simulink model "Experiment_134_cs"  (Simulink 10.1)
settings: Solver=ode8  StartTime=0.0  StopTime=20  FixedStep=1/10  RelTol=1e-3
PreLoadFcn:
  | mbxruntime.callbacks.PreLoadFcn(bdroot);
PostLoadFcn:
  | mbxruntime.callbacks.PostLoadFcn(bdroot);
InitFcn:
  | mbxruntime.callbacks.InitFcn(bdroot);
StartFcn:
  | mbxruntime.callbacks.StartFcn(bdroot);
StopFcn:
  | mbxruntime.callbacks.StopFcn(bdroot);
undefined symbols (not defined in the file or in its folder): acce_1, acce_2, acce_3, brake, steer, steer_1, steer_2, steer_3, t0_1, t0_2, t0_3, throttle, v_1, v_2, v_3, v_4
libraries: simulink x79, simulink_extras x12, PreScanSimulinkLibrary x8
(part 2 of 9)

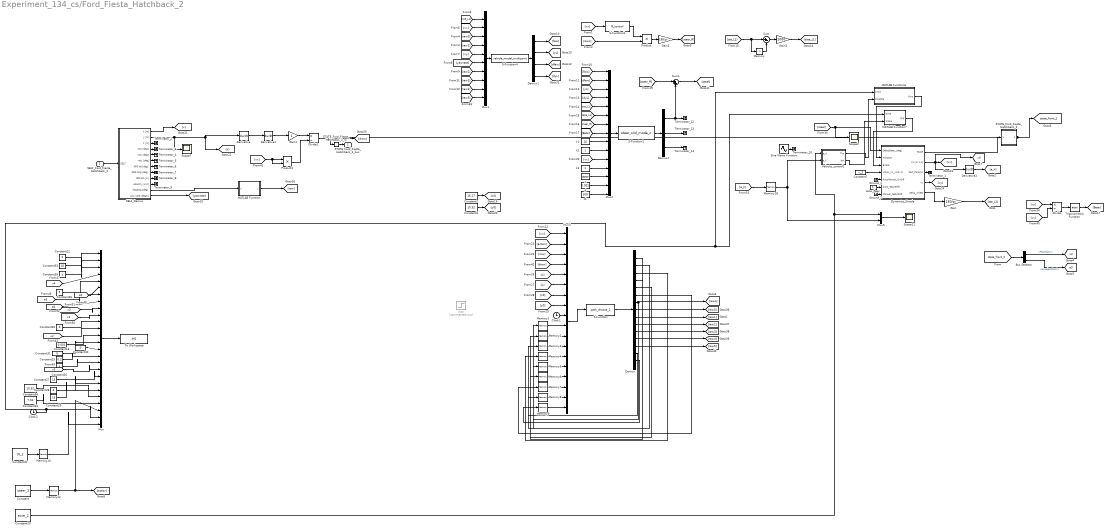
== system Experiment_134_cs/Ford_Fiesta_Hatchback_2 ==
  SELF_Ford_Fiesta_Hatchback_2 : Inport  Tag=inport/SelfPort  OutDataTypeStr=Bus: PRESCAN_SELFSENSORDATA  PortDimensions=1  SampleTime=1/10  BusOutputAsStruct=on
  Auto_Gear : Constant  Tag=AutoGear
  Bus Selector : BusSelector  OutputSignals=PositionX,AccelerationX
  Clock1 : Clock
  Clock2 : Clock
  Constant : Constant  Value=steer_2
  Constant18 : Constant  Value=0.001
  Constant2 : Constant  Value=16.27
  Constant20 : Constant  Value=acce_2
  Constant21 : Constant  Value=t0_2
  Constant22 : Constant  Value=3
  Constant25 : Constant  Value=0.2
  Constant26 : Constant  Value=6
  Constant27 : Constant  Value=15
  Constant28 : Constant  Value=4
  Constant29 : Constant  Value=15
  Constant3 : Constant  Value=10.52
  Constant30 : Constant  Value=0
  Constant31 : Constant  Value=0
  Constant32 : Constant  Value=7.04
  Constant33 : Constant  Value=10
  Constant34 : Constant  Value=10.52
  Constant35 : Constant
  Constant36 : Constant  Value=5
  Constant40 : Constant  Value=0
  Constant7 : Constant  Value=v_3
  Demux : Demux  Outputs=15
  Demux1 : Demux
  Demux2 : Demux  Outputs=3
  Derivative : Derivative
  Derivative1 : Derivative
  Derivative2 : Derivative
  Divide : Product  Inputs=*/
  Divide1 : Product  Inputs=*/
  Dynamics_Simple : Subsystem  Tag=Simple_Vehicle_Dynamics  mask(PreScan Block: Simple Dynamics){Migrate=on, TimeStep=1/10, ComputationMode=Continuous_Time}
      mask prompts: Migrate "Migrate. During migration this block will be replaced by a newer one."; TimeStep "Auto assigned: Time Step [s]"; ComputationMode "Computation mode:"
      mask help:
      | The Simple Dynamics Model is selected in the GUI to simulate vehicle dynamics behavior.
      |
      | The Simple Dynamics Model is completely open to the user. The parameters of this model can be set in the Simple Dynamics dialog in the GUI.
      |
      | For more information, please click Help.
      mask init:
      | p = SimpleDyn_pars;
      settings: DeleteFcn=PreScanBlockDeleteFcn;
      mask Help: eval('openHelp(220)')
      mask Display:
      | image(imread('SimpleDyn.png'))
      | port_label('input', 1, '{\delta}_S_t_ _e_e_r [deg]','texmode','on')
      | port_label('input', 2, 'Throttle [%]')
      | port_label('input', 3, 'Brake Pres [bar]')
      | port_label('input', 4, 'V_0 [ms-1]','texmode','on')
      | port_label('input', 5, 'Auto=[0]/Manual=[1]')
      | port_label('input', 6, 'Auto_GearShift')
      | port_label('input', 7, 'Manual_GearShift')
      | port_label('output', 1, 'State')
      | port_label('output', 2, 'Vx [ms-1]')
      | port_label('output', 3, 'Perf Params')
  Gain : Gain  Gain=180/pi
  Gain1 : Gain
  Gain2 : Gain  Gain=180/pi
  Gain3 : Gain  Gain=1000
  Ground_1 : Ground
  Ground_2 : Ground
  MATLAB Function : MATLAB Function  TreatAsAtomicUnit=on
  MATLAB Function6 : MATLAB Function  TreatAsAtomicUnit=on
  MATLAB Function7 : MATLAB Function  TreatAsAtomicUnit=on
  Memory{,1..9,18} (11 alike) : Memory
  Memory10 : Memory  InitialCondition=-3
  Memory12 : Memory  InitialCondition=10.52
  Mux : Mux  Inputs=26
  Mux1 : Mux  Inputs=10
  Mux2 : Mux  Inputs=15
  Mux3 : Mux  Inputs=18
  Mux5 : Mux  Inputs=2
  Product : Product
  Product1 : Product
  S-Function : S-Function  FunctionName=path_choose_2  SFunctionDeploymentMode=off  EnableBusSupport=off
  S-Function1 : S-Function  FunctionName=steer_slid_mode_c  SFunctionDeploymentMode=off  EnableBusSupport=off
  S-Function3 : S-Function  FunctionName=ff_control  SFunctionDeploymentMode=off  EnableBusSupport=off
  S-Function4 : S-Function  FunctionName=vehicle_model_multipoint  SFunctionDeploymentMode=off  EnableBusSupport=off
  SELF_Demux : Subsystem  Tag=demux/SelfPort  mask(PreScan Demux Block:){}
      mask help:
      | The SELF port shows (state) information of the actor itself. The outputs are position in the experiment's axis system and the GPS coordinates, and the object's absolute velocity and compass heading.
      |
      | For more information, please click Help.
      settings: DeleteFcn=PreScanBlockDeleteFcn;
      mask Help: eval('openHelp(462)')
      mask Display:
      | port_label('output',1,'x [m]')
      | port_label('output',2,'y [m]')
      | port_label('output',3,'z [m]','texmode','on')
      | port_label('output',4,'Rotx [deg]','texmode','on')
      | port_label('output',5,'Roty [deg]','texmode','on')
      | port_label('output',6,'Rotz [deg]','texmode','on')
      | port_label('output',7,'GPS lat [deg]','texmode','on')
      | port_label('output',8,'GPS long [deg]','texmode','on')
      | port_label('output',9,'GPS alt [m]','texmode','on')
      | port_label('output',10,'Velocity [m/s]')
      | port_label('output',11,'Heading [deg]')
      | port_label('output',12,'Yaw rate [deg/s]')
  STATE_Ford_Fiesta_Hatchback_2 : Subsystem  Tag=mux/StatePort  Priority=0  LoadFcn=load PrescanStateActuatorData  mask(PreScan Sink Block: State){x0=12.8194, y0=10.3324, z0=0.5, Roll0=0, Pitch0=0, Yaw0=0, TimeStep=1/10}
      mask prompts: x0 "Ini x-position VEHICLE wrt GLOBAL axis system [m]"; y0 "Ini y-position VEHICLE wrt GLOBAL axis system [m]"; z0 "Ini z-position VEHICLE wrt GLOBAL axis system [m]"; Roll0 "Ini roll-angle BODY wrt VEHICLE axis system [deg]"; Pitch0 "Ini pitch-angle BODY wrt VEHICLE axis system [deg]"; Yaw0 "Ini yaw-angle VEHICLE wrt GLOBAL axis system [deg]"; TimeStep "Auto-Assigned: Upload Period [s]"
      mask help:
      | The Actor State contains a vector signal of size (9x1), containing the following signals:
      |
      | -  Position                  (x,y,z)                                     [m]
      | -  Velocity                  (vx,vy,vz)                               [m/s]
      | -  Angles                    (Roll, Pitch, Yaw)                   [rad]
      |
      | The Actor state is defined in the global axis system.
      | The state is superponed on the Initial position defined in the GUI.
      |
      | For more information, please click Help.
      settings: DeleteFcn=PreScanBlockDeleteFcn;
      mask Help: eval('openHelp(222)')
      mask Display: image(imread('State.png'))
  STATE_Ford_Fiesta_Hatchback_2_rc : RateTransition  Tag=mux_rc/StatePort  OutPortSampleTimeOpt=Inherit
  Scope11 : Scope
  Scope2 : Scope
  Scope7 : Scope
  Sine Wave Function : Sin  SampleTime=0
  Step : Step  Commented=on  Time=2  Before=10.52  After=7.04  SampleTime=0
  Sum : Sum  Inputs=|+-
  Sum1 : Sum  Inputs=|++
  Terminator_{1..10,12..14} (13 alike) : Terminator
  To Workspace : ToWorkspace  VariableName=IM2  SampleTime=-1
      settings: MaxDataPoints=1  Save2DSignal=2-D array (concatenate along first dimension)
  Trigonometric Function : Trigonometry  Operator=atan
  Velocity_control1 : Subsystem
  c : Constant  Value=18000
  c1 : Constant  Value=100
  d : Constant  Value=0.001
  k1 : Constant  Value=20
  k2 : Constant
  k3 : Constant
  STATE_Ford_Fiesta_Hatchback_2_bus : Outport  Tag=outport/StatePort  OutDataTypeStr=Bus: PRESCAN_STATEACTUATORDATA  PortDimensions=1  SampleTime=1/10
  tag scope: a3=global, state_front_2=global, v3=global, x3=global
  wires:
  STATE_Ford_Fiesta_Hatchback_2/1(StateBus) -> [state_front_2], STATE_Ford_Fiesta_Hatchback_2_rc/1
  [steel] -> Dynamics_Simple/1(DeltaSteer_[deg]), Scope2/1
  Velocity_control1/1(Tho) -> MATLAB Function6/2(throttle)
  Velocity_control1/2(brk) -> MATLAB Function7/2(brake)
  Constant7/1 -> Dynamics_Simple/4(Initial_Vx_[ms-1])
  SELF_Demux/1(x [m]) -> [x]
  SELF_Demux/12(yaw rate [deg/s]) -> [yawrate]
  SELF_Demux/11(heading [deg]) -> MATLAB Function/1(u)
  Derivative/1 -> Derivative1/1
  MATLAB Function/1(y) -> [row]
  Gain1/1 -> Divide1/1
  Derivative1/1 -> Gain1/1
  Product1/1 -> Divide1/2
  SELF_Demux/2(y [m]) -> Scope7/1, [y], Derivative/1
  [vx] -> Product1/2, Product1/1
  Divide1/1 -> [drow]
  [ste_L1] -> Memory/1, Sum/1
  S-Function4/1 -> Demux1/1
  [raw0] -> Mux1/3
  Demux1/3 -> [dfaio]
  [dyL] -> Mux2/4
  Mux2/1 -> S-Function1/1
  [dfaio] -> Mux2/2
  Product/1 -> Gain2/1
  Gain3/1 -> [dste_L1]
  c/1 -> Mux2/13
  Mux1/1 -> S-Function4/1
  [raw2] -> Mux1/7
  [raw1] -> Mux1/4
  [yawrate] -> Mux1/6
  k1/1 -> Mux2/9
  [steer_ff] -> Sum1/1
  [raw4] -> Mux1/9
  S-Function3/1 -> Product/1
  k2/1 -> Mux2/10
  Sum1/1 -> [steel]
  k3/1 -> Mux2/12
  [vy] -> Mux1/5
  Demux2/1 -> Terminator_12/1, Sum1/2
  Demux1/2 -> [yL]
  [rawL] -> Product/2
  [yL] -> Mux2/3
  Demux1/1 -> [faio]
  [Beta] -> Mux2/8
  Sum/1 -> Gain3/1
  c1/1 -> Mux2/15
  Memory/1 -> Sum/2
  [ste_L1] -> Mux1/1
  Demux1/4 -> [dyL]
  Demux2/2 -> Terminator_13/1
  [raw3] -> Mux1/8
  [vx] -> S-Function3/1
  Gain2/1 -> [steer_ff]
  [steer_ff] -> Mux2/7
  [vx] -> Mux2/11
  d/1 -> Mux2/14
  [vx] -> Mux1/2
  [ste_L1] -> Mux2/5
  [faio] -> Mux2/1
  Demux2/3 -> Terminator_14/1
  [raw5] -> Mux1/10
  [dste_L1] -> Mux2/6
  S-Function1/1 -> Demux2/1
  Constant3/1 -> [y0]
  Constant2/1 -> [x0]
  Mux5/1 -> Scope11/1
  [row] -> Mux3/3
  [y0] -> Mux3/8
  Memory2/1 -> Mux3/11
  Memory4/1 -> Mux3/13
  Demux/15 -> Memory9/1
  Demux/13 -> [raw5]
  Memory8/1 -> Mux3/17
  Demux/8 -> [raw0]
  Clock1/1 -> Mux3/9
  Demux/9 -> [raw1]
  Memory9/1 -> Mux3/18
  Demux/12 -> [raw4]
  Demux/14 -> Memory8/1
  Memory5/1 -> Mux3/14
  Demux/7 -> [rawL], Memory1/1
  Demux/6 -> Memory7/1
  Demux/10 -> [raw2]
  Memory7/1 -> Mux3/16
  Demux/3 -> Memory4/1
  [y] -> Mux3/6
  Demux/2 -> Memory3/1
  Memory6/1 -> Mux3/15
  Memory1/1 -> Mux3/10
  Memory3/1 -> Mux3/12
  Demux/4 -> Memory5/1
  Demux/5 -> Memory6/1
  [x] -> Mux3/5
  Demux/1 -> Memory2/1
  [vx] -> Mux3/1
  [action] -> Mux3/2
  S-Function/1 -> Demux/1
  [drow] -> Mux3/4
  Mux3/1 -> S-Function/1
  [x0] -> Mux3/7
  Demux/11 -> [raw3]
  Divide/1 -> Trigonometric Function/1
  [vy] -> Divide/1
  [vx] -> Divide/2
  Dynamics_Simple/2(Vx [m s-1]) -> [v3], Derivative2/1, [vx]
  Trigonometric Function/1 -> [Beta]
  Gain/1 -> [ste_L1]
  Derivative2/1 -> [a_h]
  Dynamics_Simple/4(vy) -> [vy]
  Dynamics_Simple/5(delta_wheel) -> Gain/1
  Bus Selector/1 -> [x3]  "<PositionX>"
  [state_front_2] -> Bus Selector/1
  Bus Selector/2 -> [a3]  "<AccelerationX>"
  [a_h] -> Memory18/1
  Memory18/1 -> Mux5/2, Velocity_control1/2(a_t)
  MATLAB Function6/1(thro) -> Dynamics_Simple/2(Throttle)
  MATLAB Function7/1(bra) -> Dynamics_Simple/3(Brake)
  Constant28/1 -> Mux/20
  Constant29/1 -> Mux/21
  Clock2/1 -> Mux/25, MATLAB Function7/1(time), MATLAB Function6/1(time)
  Constant26/1 -> Mux/17
  Constant25/1 -> Mux/16
  Constant27/1 -> Mux/19
  Constant35/1 -> Mux/3
  [a3] -> Mux/7
  Mux/1 -> To Workspace/1
  Memory10/1 -> Mux/26
  Constant31/1 -> Mux/14
  Constant18/1 -> Mux/13
  [v3] -> Mux/18
  Constant21/1 -> Memory10/1
  Memory12/1 -> [action], Mux/24
  Constant22/1 -> Mux/1
  Constant36/1 -> Mux/5
  [a2] -> Mux/6
  Constant33/1 -> Mux/2
  [v2] -> Mux/12
  Constant30/1 -> Mux/11
  [v4] -> Mux/4
  Constant/1 -> Memory12/1
  Constant40/1 -> Mux/15
  [a4] -> Mux/8
  Constant34/1 -> Mux/22
  Constant32/1 -> Mux/23
  Constant20/1 -> Velocity_control1/1(a_d), Mux5/1
  [x3] -> Mux/9
  [x4] -> Mux/10
  STATE_Ford_Fiesta_Hatchback_2_rc/1 -> STATE_Ford_Fiesta_Hatchback_2_bus/1
  SELF_Ford_Fiesta_Hatchback_2/1 -> SELF_Demux/1(SELF)
  Auto_Gear/1 -> Dynamics_Simple/6(Auto_GearShift)
  Dynamics_Simple/1(State) -> STATE_Ford_Fiesta_Hatchback_2/1(State)
  Ground_1/1 -> Dynamics_Simple/5(AutoManual_OnOff)
  Ground_2/1 -> Dynamics_Simple/7(Manual_GearShift)
  Dynamics_Simple/3(Perf_Params) -> Terminator_1/1
  SELF_Demux/3(z [m]) -> Terminator_2/1
  SELF_Demux/4(rotx [deg]) -> Terminator_3/1
  SELF_Demux/5(roty [deg]) -> Terminator_4/1
  SELF_Demux/6(rotz [deg]) -> Terminator_5/1
  SELF_Demux/7(GPS lat [deg]) -> Terminator_6/1
  SELF_Demux/8(GPS long [deg]) -> Terminator_7/1
  SELF_Demux/9(GPS alt [m]) -> Terminator_8/1
  SELF_Demux/10(velocity [m/s]) -> Terminator_9/1
  Sine Wave Function/1 -> Terminator_10/1

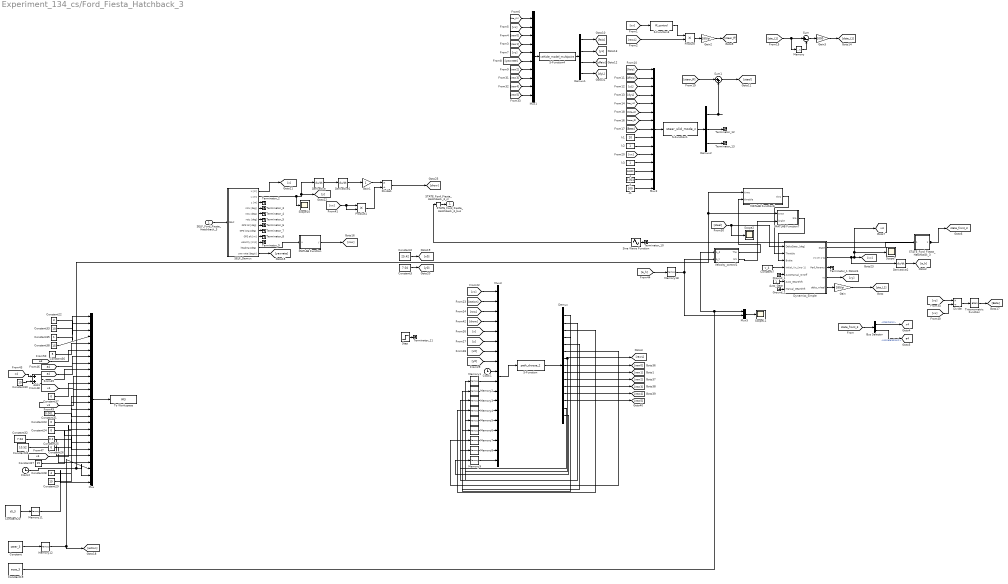
== system Experiment_134_cs/Ford_Fiesta_Hatchback_3 ==
  SELF_Ford_Fiesta_Hatchback_3 : Inport  Tag=inport/SelfPort  OutDataTypeStr=Bus: PRESCAN_SELFSENSORDATA  PortDimensions=1  SampleTime=1/10  BusOutputAsStruct=on
  Add1 : Sum
  Auto_Gear : Constant  Tag=AutoGear
  Bus Selector : BusSelector  OutputSignals=PositionX,AccelerationX
  Clock1 : Clock
  Clock2 : Clock
  Constant : Constant  Value=steer_3
  Constant19 : Constant  Value=acce_3
  Constant2 : Constant  Value=25.42
  Constant20 : Constant  Value=t0_3
  Constant22 : Constant  Value=3
  Constant23 : Constant  Value=0
  Constant24 : Constant  Value=0
  Constant25 : Constant  Value=0.2
  Constant26 : Constant  Value=6
  Constant{27,29..30,38} (4 alike) : Constant  Value=15
  Constant28 : Constant  Value=4
  Constant3 : Constant  Value=7.04
  Constant31 : Constant  Value=0.001
  Constant32 : Constant  Value=7.04
  Constant33 : Constant  Value=10
  Constant34 : Constant  Value=10.52
  Constant35 : Constant
  Constant36 : Constant  Value=5
  Constant37 : Constant  Value=0
  Constant7 : Constant  Value=v_4
  Demux : Demux  Outputs=15
  Demux1 : Demux
  Demux2 : Demux  Outputs=3
  Derivative : Derivative
  Derivative1 : Derivative
  Derivative2 : Derivative
  Divide : Product  Inputs=*/
  Divide1 : Product  Inputs=*/
  Dynamics_Simple : Subsystem  Tag=Simple_Vehicle_Dynamics  mask(PreScan Block: Simple Dynamics){Migrate=on, TimeStep=1/10, ComputationMode=Continuous_Time}
      mask prompts: Migrate "Migrate. During migration this block will be replaced by a newer one."; TimeStep "Auto assigned: Time Step [s]"; ComputationMode "Computation mode:"
      mask help:
      | The Simple Dynamics Model is selected in the GUI to simulate vehicle dynamics behavior.
      |
      | The Simple Dynamics Model is completely open to the user. The parameters of this model can be set in the Simple Dynamics dialog in the GUI.
      |
      | For more information, please click Help.
      mask init:
      | p = SimpleDyn_pars;
      settings: DeleteFcn=PreScanBlockDeleteFcn;
      mask Help: eval('openHelp(220)')
      mask Display:
      | image(imread('SimpleDyn.png'))
      | port_label('input', 1, '{\delta}_S_t_ _e_e_r [deg]','texmode','on')
      | port_label('input', 2, 'Throttle [%]')
      | port_label('input', 3, 'Brake Pres [bar]')
      | port_label('input', 4, 'V_0 [ms-1]','texmode','on')
      | port_label('input', 5, 'Auto=[0]/Manual=[1]')
      | port_label('input', 6, 'Auto_GearShift')
      | port_label('input', 7, 'Manual_GearShift')
      | port_label('output', 1, 'State')
      | port_label('output', 2, 'Vx [ms-1]')
      | port_label('output', 3, 'Perf Params')
  Gain : Gain  Gain=180/pi
  Gain1 : Gain
  Gain2 : Gain  Gain=180/pi
  Gain3 : Gain  Gain=1000
  Ground_1 : Ground
  Ground_2 : Ground
  MATLAB Function : MATLAB Function  TreatAsAtomicUnit=on
  MATLAB Function6 : MATLAB Function  TreatAsAtomicUnit=on
  MATLAB Function7 : MATLAB Function  TreatAsAtomicUnit=on
  Memory{,1..9,18} (11 alike) : Memory
  Memory11 : Memory  InitialCondition=-3
  Memory12 : Memory  InitialCondition=7.04
  Mux : Mux  Inputs=26
  Mux1 : Mux  Inputs=10
  Mux2 : Mux  Inputs=15
  Mux3 : Mux  Inputs=18
  Mux5 : Mux  Inputs=2
  Product : Product
  Product1 : Product
  S-Function : S-Function  FunctionName=path_choose_2  SFunctionDeploymentMode=off  EnableBusSupport=off
  S-Function1 : S-Function  FunctionName=steer_slid_mode_c  SFunctionDeploymentMode=off  EnableBusSupport=off
  S-Function3 : S-Function  FunctionName=ff_control  SFunctionDeploymentMode=off  EnableBusSupport=off
  S-Function4 : S-Function  FunctionName=vehicle_model_multipoint  SFunctionDeploymentMode=off  EnableBusSupport=off
  SELF_Demux : Subsystem  Tag=demux/SelfPort  mask(PreScan Demux Block:){}
      mask help:
      | The SELF port shows (state) information of the actor itself. The outputs are position in the experiment's axis system and the GPS coordinates, and the object's absolute velocity and compass heading.
      |
      | For more information, please click Help.
      settings: DeleteFcn=PreScanBlockDeleteFcn;
      mask Help: eval('openHelp(462)')
      mask Display:
      | port_label('output',1,'x [m]')
      | port_label('output',2,'y [m]')
      | port_label('output',3,'z [m]','texmode','on')
      | port_label('output',4,'Rotx [deg]','texmode','on')
      | port_label('output',5,'Roty [deg]','texmode','on')
      | port_label('output',6,'Rotz [deg]','texmode','on')
      | port_label('output',7,'GPS lat [deg]','texmode','on')
      | port_label('output',8,'GPS long [deg]','texmode','on')
      | port_label('output',9,'GPS alt [m]','texmode','on')
      | port_label('output',10,'Velocity [m/s]')
      | port_label('output',11,'Heading [deg]')
      | port_label('output',12,'Yaw rate [deg/s]')
  STATE_Ford_Fiesta_Hatchback_3 : Subsystem  Tag=mux/StatePort  Priority=0  LoadFcn=load PrescanStateActuatorData  mask(PreScan Sink Block: State){x0=29.1805, y0=6.9131, z0=0.5, Roll0=0, Pitch0=0, Yaw0=0, TimeStep=1/10}
      mask prompts: x0 "Ini x-position VEHICLE wrt GLOBAL axis system [m]"; y0 "Ini y-position VEHICLE wrt GLOBAL axis system [m]"; z0 "Ini z-position VEHICLE wrt GLOBAL axis system [m]"; Roll0 "Ini roll-angle BODY wrt VEHICLE axis system [deg]"; Pitch0 "Ini pitch-angle BODY wrt VEHICLE axis system [deg]"; Yaw0 "Ini yaw-angle VEHICLE wrt GLOBAL axis system [deg]"; TimeStep "Auto-Assigned: Upload Period [s]"
      mask help:
      | The Actor State contains a vector signal of size (9x1), containing the following signals:
      |
      | -  Position                  (x,y,z)                                     [m]
      | -  Velocity                  (vx,vy,vz)                               [m/s]
      | -  Angles                    (Roll, Pitch, Yaw)                   [rad]
      |
      | The Actor state is defined in the global axis system.
      | The state is superponed on the Initial position defined in the GUI.
      |
      | For more information, please click Help.
      settings: DeleteFcn=PreScanBlockDeleteFcn;
      mask Help: eval('openHelp(222)')
      mask Display: image(imread('State.png'))
  STATE_Ford_Fiesta_Hatchback_3_rc : RateTransition  Tag=mux_rc/StatePort  OutPortSampleTimeOpt=Inherit
  Scope{2,7,10..11} (4 alike) : Scope
  Sine Wave Function : Sin  SampleTime=0
  Step : Step  Time=2  Before=7.04  After=10.52  SampleTime=0
  Sum : Sum  Inputs=|+-
  Sum1 : Sum  Inputs=|++
  Terminator_{1..13} (13 alike) : Terminator
  To Workspace : ToWorkspace  VariableName=IM3  SampleTime=-1
      settings: MaxDataPoints=1  Save2DSignal=2-D array (concatenate along first dimension)
  Trigonometric Function : Trigonometry  Operator=atan
  Velocity_control1 : Subsystem
  c : Constant  Value=14000
  c1 : Constant  Value=100
  d : Constant  Value=0.001
  k1 : Constant  Value=20
  k2 : Constant
  k3 : Constant
  STATE_Ford_Fiesta_Hatchback_3_bus : Outport  Tag=outport/StatePort  OutDataTypeStr=Bus: PRESCAN_STATEACTUATORDATA  PortDimensions=1  SampleTime=1/10
  tag scope: a4=global, state_front_3=global, v4=global, x4=global
  wires:
  STATE_Ford_Fiesta_Hatchback_3/1(StateBus) -> [state_front_3], STATE_Ford_Fiesta_Hatchback_3_rc/1
  [steel] -> Dynamics_Simple/1(DeltaSteer_[deg]), Scope2/1
  Velocity_control1/1(Tho) -> MATLAB Function6/2(throttle)
  Velocity_control1/2(brk) -> MATLAB Function7/2(brake)
  Constant7/1 -> Dynamics_Simple/4(Initial_Vx_[ms-1])
  SELF_Demux/1(x [m]) -> [x]
  SELF_Demux/12(yaw rate [deg/s]) -> [yawrate]
  SELF_Demux/11(heading [deg]) -> MATLAB Function/1(u)
  Derivative/1 -> Derivative1/1
  MATLAB Function/1(y) -> [row]
  Gain1/1 -> Divide1/1
  Derivative1/1 -> Gain1/1
  Product1/1 -> Divide1/2
  SELF_Demux/2(y [m]) -> Scope10/1, Derivative/1, [y]
  [vx] -> Product1/2, Product1/1
  Divide1/1 -> [drow]
  [ste_L1] -> Memory/1, Sum/1
  S-Function4/1 -> Demux1/1
  [raw0] -> Mux1/3
  Demux1/3 -> [dfaio]
  [dyL] -> Mux2/4
  Mux2/1 -> S-Function1/1
  [dfaio] -> Mux2/2
  Product/1 -> Gain2/1
  Gain3/1 -> [dste_L1]
  c/1 -> Mux2/13
  Mux1/1 -> S-Function4/1
  [raw2] -> Mux1/7
  [raw1] -> Mux1/4
  [yawrate] -> Mux1/6
  k1/1 -> Mux2/9
  [steer_ff] -> Sum1/1
  [raw4] -> Mux1/9
  S-Function3/1 -> Product/1
  k2/1 -> Mux2/10
  Sum1/1 -> [steel]
  k3/1 -> Mux2/12
  [vy] -> Mux1/5
  Demux2/1 -> Sum1/2
  Demux1/2 -> [yL]
  [rawL] -> Product/2
  [yL] -> Mux2/3
  Demux1/1 -> [faio]
  [Beta] -> Mux2/8
  Sum/1 -> Gain3/1
  c1/1 -> Mux2/15
  Memory/1 -> Sum/2
  [ste_L1] -> Mux1/1
  Demux1/4 -> [dyL]
  Demux2/2 -> Terminator_12/1
  [raw3] -> Mux1/8
  [vx] -> S-Function3/1
  Gain2/1 -> [steer_ff]
  [steer_ff] -> Mux2/7
  [vx] -> Mux2/11
  d/1 -> Mux2/14
  [vx] -> Mux1/2
  [ste_L1] -> Mux2/5
  [faio] -> Mux2/1
  Demux2/3 -> Terminator_13/1
  [raw5] -> Mux1/10
  [dste_L1] -> Mux2/6
  S-Function1/1 -> Demux2/1
  [row] -> Mux3/3
  [y0] -> Mux3/8
  Memory2/1 -> Mux3/11
  Memory4/1 -> Mux3/13
  Demux/15 -> Memory9/1
  Demux/13 -> [raw5]
  Memory8/1 -> Mux3/17
  Demux/8 -> [raw0]
  Clock1/1 -> Mux3/9
  Demux/9 -> [raw1]
  Memory9/1 -> Mux3/18
  Demux/12 -> [raw4]
  Demux/14 -> Memory8/1
  Memory5/1 -> Mux3/14
  Demux/7 -> [rawL], Memory1/1
  Demux/6 -> Memory7/1
  Demux/10 -> [raw2]
  Memory7/1 -> Mux3/16
  Demux/3 -> Memory4/1
  [y] -> Mux3/6
  Demux/2 -> Memory3/1
  Memory6/1 -> Mux3/15
  Memory1/1 -> Mux3/10
  Memory3/1 -> Mux3/12
  Demux/4 -> Memory5/1
  Demux/5 -> Memory6/1
  [x] -> Mux3/5
  Demux/1 -> Memory2/1
  [vx] -> Mux3/1
  [action] -> Mux3/2
  S-Function/1 -> Demux/1
  [drow] -> Mux3/4
  Mux3/1 -> S-Function/1
  [x0] -> Mux3/7
  Demux/11 -> [raw3]
  Constant3/1 -> [y0]
  Constant2/1 -> [x0]
  Mux5/1 -> Scope11/1
  Dynamics_Simple/4(vy) -> [vy]
  [vy] -> Divide/1
  [vx] -> Divide/2
  Trigonometric Function/1 -> [Beta]
  Gain/1 -> [ste_L1]
  Derivative2/1 -> [a_h]
  Divide/1 -> Trigonometric Function/1
  Dynamics_Simple/2(Vx [m s-1]) -> Derivative2/1, [v4], Scope7/1, [vx]
  Dynamics_Simple/5(delta_wheel) -> Gain/1
  Bus Selector/1 -> [x4]  "<PositionX>"
  [state_front_3] -> Bus Selector/1
  Bus Selector/2 -> [a4]  "<AccelerationX>"
  [a_h] -> Memory18/1
  Memory18/1 -> Mux5/2, Velocity_control1/2(a_t)
  MATLAB Function7/1(bra) -> Dynamics_Simple/3(Brake)
  MATLAB Function6/1(thro) -> Dynamics_Simple/2(Throttle)
  Add1/1 -> Mux/9
  Constant30/1 -> Add1/2
  [a3] -> Mux/6
  [x4] -> Add1/1
  Constant22/1 -> Mux/1
  Constant33/1 -> Mux/2
  Constant35/1 -> Mux/3
  Constant38/1 -> Mux/4
  Constant36/1 -> Mux/5
  [a4] -> Mux/7
  [a4] -> Mux/8
  [x4] -> Mux/10
  Constant37/1 -> Mux/11
  [v3] -> Mux/12
  Constant31/1 -> Mux/13
  Constant23/1 -> Mux/14
  Constant24/1 -> Mux/15
  Constant25/1 -> Mux/16
  Constant26/1 -> Mux/17
  [v4] -> Mux/18
  Constant27/1 -> Mux/19
  Constant28/1 -> Mux/20
  Constant29/1 -> Mux/21
  Constant32/1 -> Mux/22
  Constant34/1 -> Mux/23
  Clock2/1 -> MATLAB Function6/1(time), MATLAB Function7/1(time), Mux/25
  Constant20/1 -> Memory11/1
  Memory11/1 -> Mux/26
  Mux/1 -> To Workspace/1
  Constant/1 -> Memory12/1
  Constant19/1 -> Velocity_control1/1(a_d), Mux5/1
  Memory12/1 -> [action], Mux/24
  STATE_Ford_Fiesta_Hatchback_3_rc/1 -> STATE_Ford_Fiesta_Hatchback_3_bus/1
  SELF_Ford_Fiesta_Hatchback_3/1 -> SELF_Demux/1(SELF)
  Auto_Gear/1 -> Dynamics_Simple/6(Auto_GearShift)
  Dynamics_Simple/1(State) -> STATE_Ford_Fiesta_Hatchback_3/1(State)
  Ground_1/1 -> Dynamics_Simple/5(AutoManual_OnOff)
  Ground_2/1 -> Dynamics_Simple/7(Manual_GearShift)
  Dynamics_Simple/3(Perf_Params) -> Terminator_1/1
  SELF_Demux/3(z [m]) -> Terminator_2/1
  SELF_Demux/4(rotx [deg]) -> Terminator_3/1
  SELF_Demux/5(roty [deg]) -> Terminator_4/1
  SELF_Demux/6(rotz [deg]) -> Terminator_5/1
  SELF_Demux/7(GPS lat [deg]) -> Terminator_6/1
  SELF_Demux/8(GPS long [deg]) -> Terminator_7/1
  SELF_Demux/9(GPS alt [m]) -> Terminator_8/1
  SELF_Demux/10(velocity [m/s]) -> Terminator_9/1
  Sine Wave Function/1 -> Terminator_10/1
  Step/1 -> Terminator_11/1

== system Experiment_134_cs/PreScanTerminator ==
  Terminator : Terminator
  sfun_Terminator : S-Function  FunctionName=sfun_Terminator  Parameters=SampleTime  SFunctionDeploymentMode=off  EnableBusSupport=off  mask(Legacy Function){SFunctionSpec=void prescan_terminator_outputFcn(void ** work1, PRESCAN_TERMINATORDATA y1[1]), SampleTime=TimeStep, ShowSpec=on}
      mask prompts: SampleTime "Sample time (-1 for inherited):"; ShowSpec "Display function specification"
      mask help:
      | This block allows you to call the legacy functions specified by the following Legacy Code Tool definition:
      | def.SFunctionName = 'sfun_Terminator';
      | def.OutputFcnSpec = 'void prescan_terminator_outputFcn(void ** work1, PRESCAN_TERMINATORDATA y1[1])';
      | def.StartFcnSpec = 'void prescan_terminator_startFcn(void ** work1)';
      | def.TerminateFcnSpec = 'void prescan_terminator_terminateFcn(void ** work1)';
      | def.HeaderFiles = {'prescan_terminator_data.h'};
      | def.HostLibFiles = {'sensorinterfaced.lib'};
      | def.IncPaths = {'src', 'C:\prescandev\vislibrary\vis\..\pimp\include\sensors\InterfaceRTW'};
      | def.SrcPaths = {'src'};
      | def.LibPaths = {'C:\\prescandev\\vislibrary_build\lib'};
      | def.SampleTime = 'parameterized';
      | def.Options.language = 'C';
      mask Help: <p>This block was generated automatically by the Legacy Code Tool. For detailed help on this tool, call<a href="matlab:legacy_code('help')"> legacy_code('help')</a>.</p>
      mask Callback ShowSpec:
      | if strcmp(get_param(gcbh, 'ShowSpec'), 'on')
      |   set_param(gcbh, 'MaskDisplay', sprintf('fprintf(''%s'');', get_param(gcbh, 'SFunctionSpec')));
      | else
      |   set_param(gcbh, 'MaskDisplay', sprintf('fprintf(''%s'');', get_param(gcbh, 'FunctionName')));
      | end
      mask Display: fprintf('void prescan_terminator_outputFcn(void ** work1, PRESCAN_TERMINATORDATA y1[1])');
  wires:
  sfun_Terminator/1 -> Terminator/1

== system Experiment_134_cs/SELF_BMW_Z3_Convertible_1 ==
  Sensor : S-Function  FunctionName=sfun_SelfSensor  Parameters=UniqueID, TimeStep  SFunctionDeploymentMode=off  EnableBusSupport=off  mask(PreScan Source Block: SELF){UniqueID=511, TimeStep=1/10}
      mask prompts: UniqueID "Auto-Assigned: Unique ID"; TimeStep "Auto-Assigned: Upload Period [s]"
      mask help:
      | The SELF port shows (state) information of the actor itself. The outputs are position in the experiment's axis system and the GPS coordinates, and the object's absolute velocity and compass heading.
      |
      | For more information, please click Help.
      mask Help: eval('openHelp(462)')
      mask Display: image(imread('GPS.png'))
  SELF_BMW_Z3_Convertible_1 : Outport  Tag=outport/SelfPort  OutDataTypeStr=Bus: PRESCAN_SELFSENSORDATA  PortDimensions=1  SampleTime=1/10
  wires:
  Sensor/1 -> SELF_BMW_Z3_Convertible_1/1

== system Experiment_134_cs/SELF_Ford_Fiesta_Hatchback_1 ==
  Sensor : S-Function  FunctionName=sfun_SelfSensor  Parameters=UniqueID, TimeStep  SFunctionDeploymentMode=off  EnableBusSupport=off  mask(PreScan Source Block: SELF){UniqueID=405, TimeStep=1/10}
      mask prompts: UniqueID "Auto-Assigned: Unique ID"; TimeStep "Auto-Assigned: Upload Period [s]"
      mask help:
      | The SELF port shows (state) information of the actor itself. The outputs are position in the experiment's axis system and the GPS coordinates, and the object's absolute velocity and compass heading.
      |
      | For more information, please click Help.
      mask Help: eval('openHelp(462)')
      mask Display: image(imread('GPS.png'))
  SELF_Ford_Fiesta_Hatchback_1 : Outport  Tag=outport/SelfPort  OutDataTypeStr=Bus: PRESCAN_SELFSENSORDATA  PortDimensions=1  SampleTime=1/10
  wires:
  Sensor/1 -> SELF_Ford_Fiesta_Hatchback_1/1

== system Experiment_134_cs/SELF_Ford_Fiesta_Hatchback_2 ==
  Sensor : S-Function  FunctionName=sfun_SelfSensor  Parameters=UniqueID, TimeStep  SFunctionDeploymentMode=off  EnableBusSupport=off  mask(PreScan Source Block: SELF){UniqueID=485, TimeStep=1/10}
      mask prompts: UniqueID "Auto-Assigned: Unique ID"; TimeStep "Auto-Assigned: Upload Period [s]"
      mask help:
      | The SELF port shows (state) information of the actor itself. The outputs are position in the experiment's axis system and the GPS coordinates, and the object's absolute velocity and compass heading.
      |
      | For more information, please click Help.
      mask Help: eval('openHelp(462)')
      mask Display: image(imread('GPS.png'))
  SELF_Ford_Fiesta_Hatchback_2 : Outport  Tag=outport/SelfPort  OutDataTypeStr=Bus: PRESCAN_SELFSENSORDATA  PortDimensions=1  SampleTime=1/10
  wires:
  Sensor/1 -> SELF_Ford_Fiesta_Hatchback_2/1

== system Experiment_134_cs/SELF_Ford_Fiesta_Hatchback_3 ==
  Sensor : S-Function  FunctionName=sfun_SelfSensor  Parameters=UniqueID, TimeStep  SFunctionDeploymentMode=off  EnableBusSupport=off  mask(PreScan Source Block: SELF){UniqueID=486, TimeStep=1/10}
      mask prompts: UniqueID "Auto-Assigned: Unique ID"; TimeStep "Auto-Assigned: Upload Period [s]"
      mask help:
      | The SELF port shows (state) information of the actor itself. The outputs are position in the experiment's axis system and the GPS coordinates, and the object's absolute velocity and compass heading.
      |
      | For more information, please click Help.
      mask Help: eval('openHelp(462)')
      mask Display: image(imread('GPS.png'))
  SELF_Ford_Fiesta_Hatchback_3 : Outport  Tag=outport/SelfPort  OutDataTypeStr=Bus: PRESCAN_SELFSENSORDATA  PortDimensions=1  SampleTime=1/10
  wires:
  Sensor/1 -> SELF_Ford_Fiesta_Hatchback_3/1

== system Experiment_134_cs/STATE_BMW_Z3_Convertible_1_bus ==
  STATE_BMW_Z3_Convertible_1_bus : Inport  Tag=inport/StatePort  OutDataTypeStr=Bus: PRESCAN_STATEACTUATORDATA  PortDimensions=1  SampleTime=1/10  BusOutputAsStruct=on
  Actuator : S-Function  FunctionName=sfun_StateActuator  Parameters=UniqueID, TimeStep  SFunctionDeploymentMode=off  EnableBusSupport=off  mask(PreScan Sink Block: State){UniqueID=511, TimeStep=1/10}
      mask prompts: UniqueID "Auto-Assigned: Unique ID"; TimeStep "Auto-Assigned: Upload Period [s]"
      mask help:
      | The Actor State contains a vector signal of size (9x1), containing the following signals:
      |
      | -  Position    	(x,y,z)             	[m]
      | -  Velocity    	(vx,vy,vz)         	[m/s]
      | -  Angles       	(Roll, Pitch, Yaw)	[rad]
      |
      | The Actor state is defined in the global axis system.
      | The state is superponed on the Initial position defined in the GUI.
      |
      | For more information, please click Help.
      mask Help: eval('openHelp(222)')
      mask Display: image(imread('State.png'))
  wires:
  STATE_BMW_Z3_Convertible_1_bus/1 -> Actuator/1

== system Experiment_134_cs/STATE_Ford_Fiesta_Hatchback_1_bus ==
  STATE_Ford_Fiesta_Hatchback_1_bus : Inport  Tag=inport/StatePort  OutDataTypeStr=Bus: PRESCAN_STATEACTUATORDATA  PortDimensions=1  SampleTime=1/10  BusOutputAsStruct=on
  Actuator : S-Function  FunctionName=sfun_StateActuator  Parameters=UniqueID, TimeStep  SFunctionDeploymentMode=off  EnableBusSupport=off  mask(PreScan Sink Block: State){UniqueID=405, TimeStep=1/10}
      mask prompts: UniqueID "Auto-Assigned: Unique ID"; TimeStep "Auto-Assigned: Upload Period [s]"
      mask help:
      | The Actor State contains a vector signal of size (9x1), containing the following signals:
      |
      | -  Position    	(x,y,z)             	[m]
      | -  Velocity    	(vx,vy,vz)         	[m/s]
      | -  Angles       	(Roll, Pitch, Yaw)	[rad]
      |
      | The Actor state is defined in the global axis system.
      | The state is superponed on the Initial position defined in the GUI.
      |
      | For more information, please click Help.
      mask Help: eval('openHelp(222)')
      mask Display: image(imread('State.png'))
  wires:
  STATE_Ford_Fiesta_Hatchback_1_bus/1 -> Actuator/1

== system Experiment_134_cs/STATE_Ford_Fiesta_Hatchback_2_bus ==
  STATE_Ford_Fiesta_Hatchback_2_bus : Inport  Tag=inport/StatePort  OutDataTypeStr=Bus: PRESCAN_STATEACTUATORDATA  PortDimensions=1  SampleTime=1/10  BusOutputAsStruct=on
  Actuator : S-Function  FunctionName=sfun_StateActuator  Parameters=UniqueID, TimeStep  SFunctionDeploymentMode=off  EnableBusSupport=off  mask(PreScan Sink Block: State){UniqueID=485, TimeStep=1/10}
      mask prompts: UniqueID "Auto-Assigned: Unique ID"; TimeStep "Auto-Assigned: Upload Period [s]"
      mask help:
      | The Actor State contains a vector signal of size (9x1), containing the following signals:
      |
      | -  Position    	(x,y,z)             	[m]
      | -  Velocity    	(vx,vy,vz)         	[m/s]
      | -  Angles       	(Roll, Pitch, Yaw)	[rad]
      |
      | The Actor state is defined in the global axis system.
      | The state is superponed on the Initial position defined in the GUI.
      |
      | For more information, please click Help.
      mask Help: eval('openHelp(222)')
      mask Display: image(imread('State.png'))
  wires:
  STATE_Ford_Fiesta_Hatchback_2_bus/1 -> Actuator/1

== system Experiment_134_cs/STATE_Ford_Fiesta_Hatchback_3_bus ==
  STATE_Ford_Fiesta_Hatchback_3_bus : Inport  Tag=inport/StatePort  OutDataTypeStr=Bus: PRESCAN_STATEACTUATORDATA  PortDimensions=1  SampleTime=1/10  BusOutputAsStruct=on
  Actuator : S-Function  FunctionName=sfun_StateActuator  Parameters=UniqueID, TimeStep  SFunctionDeploymentMode=off  EnableBusSupport=off  mask(PreScan Sink Block: State){UniqueID=486, TimeStep=1/10}
      mask prompts: UniqueID "Auto-Assigned: Unique ID"; TimeStep "Auto-Assigned: Upload Period [s]"
      mask help:
      | The Actor State contains a vector signal of size (9x1), containing the following signals:
      |
      | -  Position    	(x,y,z)             	[m]
      | -  Velocity    	(vx,vy,vz)         	[m/s]
      | -  Angles       	(Roll, Pitch, Yaw)	[rad]
      |
      | The Actor state is defined in the global axis system.
      | The state is superponed on the Initial position defined in the GUI.
      |
      | For more information, please click Help.
      mask Help: eval('openHelp(222)')
      mask Display: image(imread('State.png'))
  wires:
  STATE_Ford_Fiesta_Hatchback_3_bus/1 -> Actuator/1

== system Experiment_134_cs/Synchronizer ==
  Bus Selector1 : BusSelector  OutputSignals=FederateStopped
  Stop Simulation : Stop
  sfun_Synchronizer : S-Function  FunctionName=sfun_Synchronizer  Parameters=SampleTime  SFunctionDeploymentMode=off  EnableBusSupport=off  mask(Legacy Function){SFunctionSpec=void prescan_synchronizer_outputFcn(void ** work1, PRESCAN_SYNCHRONIZEDATA y1[1]), SampleTime=TimeStep, ShowSpec=on}
      mask prompts: SampleTime "Sample time (-1 for inherited):"; ShowSpec "Display function specification"
      mask help:
      | This block allows you to call the legacy functions specified by the following Legacy Code Tool definition:
      | def.SFunctionName = 'sfun_Synchronizer';
      | def.OutputFcnSpec = 'void prescan_synchronizer_outputFcn(void ** work1, PRESCAN_SYNCHRONIZEDATA y1[1])';
      | def.StartFcnSpec = 'void prescan_synchronizer_startFcn(void ** work1)';
      | def.TerminateFcnSpec = 'void prescan_synchronizer_terminateFcn(void ** work1)';
      | def.HeaderFiles = {'prescan_synchronizer_data.h'};
      | def.HostLibFiles = {'sensorinterfaced.lib'};
      | def.IncPaths = {'src', 'C:\prescandev\vislibrary\vis\..\pimp\include\sensors\InterfaceRTW'};
      | def.SrcPaths = {'src'};
      | def.LibPaths = {'C:\\prescandev\\vislibrary_build\lib'};
      | def.SampleTime = 'parameterized';
      | def.Options.language = 'C';
      mask Help: <p>This block was generated automatically by the Legacy Code Tool. For detailed help on this tool, call<a href="matlab:legacy_code('help')"> legacy_code('help')</a>.</p>
      mask Callback ShowSpec:
      | if strcmp(get_param(gcbh, 'ShowSpec'), 'on')
      |   set_param(gcbh, 'MaskDisplay', sprintf('fprintf(''%s'');', get_param(gcbh, 'SFunctionSpec')));
      | else
      |   set_param(gcbh, 'MaskDisplay', sprintf('fprintf(''%s'');', get_param(gcbh, 'FunctionName')));
      | end
      mask Display: fprintf('void prescan_synchronizer_outputFcn(void ** work1, PRESCAN_SYNCHRONIZEDATA y1[1])');
  wires:
  Bus Selector1/1 -> Stop Simulation/1  "<FederateStopped>"
  sfun_Synchronizer/1 -> Bus Selector1/1

== system Experiment_134_cs/BMW_Z3_Convertible_1/Dynamics_Simple ==
  DeltaSteer_[deg] : Inport
  Throttle : Inport  Port=2
  Brake : Inport  Port=3
  Initial_Vx_[ms-1] : Inport  Port=4
  AutoManual_OnOff : Inport  Port=5
  Auto_GearShift : Inport  Port=6
  Manual_GearShift : Inport  Port=7
  Bus Creator : BusCreator  Inputs=14
  Chassis : Subsystem
      mask Display: image(imread('Chassis.png'));
  Engine : Subsystem
      mask Display: image(imread('Engine.png'));
  Gain : Gain  Gain=3.6
  Gear: Auto Manual : Subsystem
  Radians to Degrees : simulink_extras/Transformations/Radians to Degrees
  Radians to Degrees1 : simulink_extras/Transformations/Radians to Degrees
  Selector : Selector  InputPortWidth=9  IndexOptions=Index vector (dialog)  Indices=7  OutputSizes=1
  Selector1 : Selector  InputPortWidth=9  IndexOptions=Index vector (dialog)  Indices=8  OutputSizes=1
  ShiftLogic : Subsystem
      mask Display: image(imread('Gearshift.png'));
  Transmission : Subsystem
      mask Display: image(imread('Transmission.png'));
  State : Outport
  Vx [m s-1] : Outport  Port=2
  Perf_Params : Outport  Port=3
  wires:
  [vy] -> Bus Creator/14  "vy_[ms-1]"
  [vx] -> Bus Creator/13  "vx_[ms-1]"
  Chassis/7(TransmissionOut_[rpm]) -> Transmission/3(n_TransmissionOut_[rpm])  "n_driveline_[rpm]"
  Chassis/6(PDrive_[kW]) -> [PD]
  Chassis/5(ay_[ms-2]) -> [ay]
  Chassis/4(ax_[ms-2]) -> [ax]
  Chassis/3(Vy_[ms-1]) -> [vy]
  [vx] -> ShiftLogic/4(VehSpeed_[ms-1])
  Gear: Auto Manual/1(Gear) -> Transmission/2(GearNr_[-]), [gear]  "gear"
  Manual_GearShift/1 -> Gear: Auto Manual/2(Manual_Gear)
  AutoManual_OnOff/1 -> Gear: Auto Manual/1(Auto_Manual), [auto_manual]
  Chassis/2(VehicleSpeed_[ms-1]) -> [vx], Vx [m s-1]/1
  Auto_GearShift/1 -> ShiftLogic/3(Auto_GearShift)
  Throttle/1 -> Engine/2(Throttle_[%]), ShiftLogic/1(Throttle_[%]), [throttle]
  Initial_Vx_[ms-1]/1 -> Chassis/4(Initial_Vx_[m s-1])
  DeltaSteer_[deg]/1 -> Chassis/3(DeltaSteer_[deg])
  Chassis/1(State) -> State/1, Selector/1, Selector1/1
  Brake/1 -> [brake], Chassis/2(BrakePressure_[bar])
  Engine/1(nEngine_[rpm]) -> [RPM], Transmission/1(nEngine_[rpm])  "nEngine_[rpm]"
  ShiftLogic/1(GearNr) -> Gear: Auto Manual/3(Auto_Gear), ShiftLogic/2(GearNr_[-])  "GearNr_[-]"
  Transmission/2(TransmissionTorque_[Nm]) -> Chassis/1(TransmissionTorque_[Nm])  "TransmissionTorque_[Nm]"
  Transmission/1(ImpellerTorque_[Nm]) -> Engine/1(ImpellerTorque_[Nm])  "ImpellerTorque_[Nm]"
  Gain/1 -> Bus Creator/1  "Vx_[kmh-1]"
  [RPM] -> Bus Creator/2  "NEngine_[rpm]"
  [gear] -> Bus Creator/3  "Gear_[-]"
  [ay] -> Bus Creator/5  "Ay_[ms-2]"
  [auto_manual] -> Bus Creator/6  "Auto_Manual_[-]"
  [throttle] -> Bus Creator/7  "Throttle_[perc]"
  [brake] -> Bus Creator/8  "Brake_[bar]"
  Engine/2(PEngine_[kW]) -> [PE]
  Bus Creator/1 -> Perf_Params/1
  [PE] -> Bus Creator/9  "PEngine_[kW]"
  Radians to Degrees/1 -> Bus Creator/11  "Roll_[deg]"
  Radians to Degrees1/1 -> Bus Creator/12  "Pitch_[deg]"
  [PD] -> Bus Creator/10  "PDrive_[kW]"
  Selector/1 -> Radians to Degrees/1
  Selector1/1 -> Radians to Degrees1/1
  [vx] -> Gain/1
  [ax] -> Bus Creator/4  "Ax_[ms-2]"

== system Experiment_134_cs/BMW_Z3_Convertible_1/Reward & Terminal ==
  y1 : Inport
  d_x1 : Inport  Port=2
  d_x2 : Inport  Port=3
  stop_signal : Inport  Port=4
  d_heading : Inport  Port=5
  v : Inport  Port=6
  a : Inport  Port=7
  d_x3 : Inport  Port=8
  heading : Inport  Port=9
  x : Inport  Port=10
  Add : Sum  Inputs=++++++++
  Constant : Constant  Value=0.5
  Gain : Gain
  Lane_center_line_r : Subsystem
  MATLAB Function : MATLAB Function  TreatAsAtomicUnit=on
  Scope{,1..4} (5 alike) : Scope
  activate : Subsystem
  comfortable : Subsystem
  limit_a : Subsystem
  limit_v : Subsystem
  shaping : Subsystem
  terminal : Subsystem
  r : Outport
  isdone : Outport  Port=2
  wires:
  Lane_center_line_r/1(r) -> Add/6
  terminal/1(r) -> Add/7
  terminal/2(is done) -> MATLAB Function/1(isdone)
  Add/1 -> Gain/1
  y1/1 -> terminal/1(y1), Lane_center_line_r/1(y1), activate/2(y)
  stop_signal/1 -> terminal/2(stop_signal)
  MATLAB Function/1(y) -> isdone/1
  d_heading/1 -> comfortable/1(d_heading)
  comfortable/1(r) -> Scope3/1, Add/3
  activate/1(r) -> Add/5, Scope4/1
  Constant/1 -> Add/8
  v/1 -> limit_v/1(v), terminal/5(v1)
  limit_v/1(r) -> Scope2/1, Add/2
  limit_a/1(r) -> Scope1/1, Add/1
  a/1 -> limit_a/1(a)
  Gain/1 -> r/1
  d_x3/1 -> terminal/3(d_x3), activate/4(d_x_3), shaping/1(d_x3)
  heading/1 -> terminal/4(heading)
  shaping/1(r) -> Add/4, Scope/1
  d_x1/1 -> activate/1(d_x_1)
  d_x2/1 -> activate/3(d_x_2)
  x/1 -> terminal/6(x)

== system Experiment_134_cs/BMW_Z3_Convertible_1/SELF_Demux ==
  SELF : Inport  OutDataTypeStr=Bus: PRESCAN_SELFSENSORDATA
  Bus Selector : BusSelector  OutputSignals=PositionX,PositionY,PositionZ,OrientationRoll,OrientationPitch,OrientationYaw,Velocity,Yaw_rate,Lat,Long,Alt
  Demux2 : Demux  Outputs=3
  Gain : Gain  Gain=180/pi
  Gain1 : Gain  Gain=180/pi
  Vector Concatenate1 : Concatenate  NumInputs=3
  compas converter : Subsystem
  x [m] : Outport
  y [m] : Outport  Port=2
  z [m] : Outport  Port=3
  rotx [deg] : Outport  Port=4
  roty [deg] : Outport  Port=5
  rotz [deg] : Outport  Port=6
  GPS lat [deg] : Outport  Port=7
  GPS long [deg] : Outport  Port=8
  GPS alt [m] : Outport  Port=9
  velocity [m/s] : Outport  Port=10
  heading [deg] : Outport  Port=11
  yaw rate [deg/s] : Outport  Port=12
  wires:
  Bus Selector/11 -> GPS alt [m]/1  "<Alt>"
  Bus Selector/10 -> GPS long [deg]/1  "<Long>"
  Bus Selector/9 -> GPS lat [deg]/1  "<Lat>"
  Bus Selector/8 -> Gain1/1  "<Yaw_rate>"
  Bus Selector/7 -> velocity [m/s]/1  "<Velocity>"
  Bus Selector/6 -> compas converter/1(rotz [rad]), Vector Concatenate1/3  "<OrientationYaw>"
  Bus Selector/5 -> Vector Concatenate1/2  "<OrientationPitch>"
  Bus Selector/4 -> Vector Concatenate1/1  "<OrientationRoll>"
  Vector Concatenate1/1 -> Gain/1
  Bus Selector/3 -> z [m]/1  "<PositionZ>"
  Bus Selector/2 -> y [m]/1  "<PositionY>"
  Bus Selector/1 -> x [m]/1  "<PositionX>"
  SELF/1 -> Bus Selector/1
  Gain/1 -> Demux2/1
  Demux2/1 -> rotx [deg]/1
  Demux2/2 -> roty [deg]/1
  Demux2/3 -> rotz [deg]/1
  compas converter/1(heading [deg]) -> heading [deg]/1
  Gain1/1 -> yaw rate [deg/s]/1

== system Experiment_134_cs/BMW_Z3_Convertible_1/STATE_BMW_Z3_Convertible_1 ==
  State : Inport  SampleTime=TimeStep
  Bus Creator : BusCreator  Inputs=15  OutDataTypeStr=Bus: PRESCAN_STATEACTUATORDATA  NonVirtualBus=on
  Demux : Demux  Outputs=15
  iniBODYAngleswrtVEH : Constant  Value=[Roll0 Pitch0 0]  SampleTime=TimeStep
  iniVEHAngleswrtGLOB : Constant  Value=[0 0 Yaw0]  SampleTime=TimeStep
  iniVEHpositionwrtGLOB : Constant  Value=[x0 y0 z0]  SampleTime=TimeStep
  state2FullState : PreScanSimulinkLibrary/state2FullState  SystemSampleTime=-1  Latency=0  AutoFrameSizeCalculation=off
  StateBus : Outport  OutDataTypeStr=Bus: PRESCAN_STATEACTUATORDATA
  wires:
  Bus Creator/1 -> StateBus/1
  State/1 -> state2FullState/1
  state2FullState/1 -> Demux/1
  iniVEHpositionwrtGLOB/1 -> state2FullState/2
  iniBODYAngleswrtVEH/1 -> state2FullState/3
  iniVEHAngleswrtGLOB/1 -> state2FullState/4
  Demux/1 -> Bus Creator/1  "PositionX"
  Demux/2 -> Bus Creator/2  "PositionY"
  Demux/3 -> Bus Creator/3  "PositionZ"
  Demux/4 -> Bus Creator/4  "VelocityX"
  Demux/5 -> Bus Creator/5  "VelocityY"
  Demux/6 -> Bus Creator/6  "VelocityZ"
  Demux/7 -> Bus Creator/7  "AccelerationX"
  Demux/8 -> Bus Creator/8  "AccelerationY"
  Demux/9 -> Bus Creator/9  "AccelerationZ"
  Demux/10 -> Bus Creator/10  "OrientationRoll"
  Demux/11 -> Bus Creator/11  "OrientationPitch"
  Demux/12 -> Bus Creator/12  "OrientationYaw"
  Demux/13 -> Bus Creator/13  "AngularVelocityRoll"
  Demux/14 -> Bus Creator/14  "AngularVelocityPitch"
  Demux/15 -> Bus Creator/15  "AngularVelocityYaw"

== system Experiment_134_cs/BMW_Z3_Convertible_1/collision safety rule ==
  x1 : Inport
  x2 : Inport  Port=2
  x3 : Inport  Port=3
  x4 : Inport  Port=4
  v1 : Inport  Port=5
  v2 : Inport  Port=6
  v3 : Inport  Port=7
  v4 : Inport  Port=8
  thro : Inport  Port=9
  bra : Inport  Port=10
  MATLAB Function12 : MATLAB Function  TreatAsAtomicUnit=on
  collision safety rule : MATLAB Function  TreatAsAtomicUnit=on
  throttle : Outport
  brake : Outport  Port=2
  wires:
  MATLAB Function12/1(d) -> collision safety rule/1(d)
  MATLAB Function12/2(d_min) -> collision safety rule/2(d_min)
  collision safety rule/1(throttle) -> throttle/1
  collision safety rule/2(brake) -> brake/1
  thro/1 -> collision safety rule/3(thro)
  bra/1 -> collision safety rule/4(bra)
  x1/1 -> MATLAB Function12/1(x1)
  x2/1 -> MATLAB Function12/2(x2)
  x3/1 -> MATLAB Function12/3(x3)
  x4/1 -> MATLAB Function12/4(x4)
  v1/1 -> MATLAB Function12/5(v1)
  v2/1 -> MATLAB Function12/6(v2)
  v3/1 -> MATLAB Function12/7(v3)
  v4/1 -> MATLAB Function12/8(v4)

== system Experiment_134_cs/Ford_Fiesta_Hatchback_1/Dynamics_Simple ==
  DeltaSteer_[deg] : Inport
  Throttle : Inport  Port=2
  Brake : Inport  Port=3
  Initial_Vx_[ms-1] : Inport  Port=4
  AutoManual_OnOff : Inport  Port=5
  Auto_GearShift : Inport  Port=6
  Manual_GearShift : Inport  Port=7
  Bus Creator : BusCreator  Inputs=14
  Chassis : Subsystem
      mask Display: image(imread('Chassis.png'));
  Engine : Subsystem
      mask Display: image(imread('Engine.png'));
  Gain : Gain  Gain=3.6
  Gear: Auto Manual : Subsystem
  Radians to Degrees : simulink_extras/Transformations/Radians to Degrees
  Radians to Degrees1 : simulink_extras/Transformations/Radians to Degrees
  Selector : Selector  InputPortWidth=9  IndexOptions=Index vector (dialog)  Indices=7  OutputSizes=1
  Selector1 : Selector  InputPortWidth=9  IndexOptions=Index vector (dialog)  Indices=8  OutputSizes=1
  ShiftLogic : Subsystem
      mask Display: image(imread('Gearshift.png'));
  Transmission : Subsystem
      mask Display: image(imread('Transmission.png'));
  State : Outport
  Vx [m s-1] : Outport  Port=2
  Perf_Params : Outport  Port=3
  Out1 : Outport  Port=4
  Out2 : Outport  Port=5
  wires:
  [vy] -> Bus Creator/14  "vy_[ms-1]"
  [vx] -> Bus Creator/13  "vx_[ms-1]"
  Chassis/7(TransmissionOut_[rpm]) -> Transmission/3(n_TransmissionOut_[rpm])  "n_driveline_[rpm]"
  Chassis/6(PDrive_[kW]) -> [PD]
  Chassis/5(ay_[ms-2]) -> [ay]
  Chassis/4(ax_[ms-2]) -> [ax]
  Chassis/3(Vy_[ms-1]) -> Out2/1, [vy]
  [vx] -> ShiftLogic/4(VehSpeed_[ms-1])
  Gear: Auto Manual/1(Gear) -> Transmission/2(GearNr_[-]), [gear]  "gear"
  Manual_GearShift/1 -> Gear: Auto Manual/2(Manual_Gear)
  AutoManual_OnOff/1 -> Gear: Auto Manual/1(Auto_Manual), [auto_manual]
  Chassis/2(VehicleSpeed_[ms-1]) -> [vx], Vx [m s-1]/1
  Auto_GearShift/1 -> ShiftLogic/3(Auto_GearShift)
  Throttle/1 -> Engine/2(Throttle_[%]), ShiftLogic/1(Throttle_[%]), [throttle]
  Initial_Vx_[ms-1]/1 -> Chassis/4(Initial_Vx_[m s-1])
  DeltaSteer_[deg]/1 -> Chassis/3(DeltaSteer_[deg])
  Chassis/1(State) -> State/1, Selector/1, Selector1/1
  Brake/1 -> [brake], Chassis/2(BrakePressure_[bar])
  Engine/1(nEngine_[rpm]) -> [RPM], Transmission/1(nEngine_[rpm])  "nEngine_[rpm]"
  ShiftLogic/1(GearNr) -> Gear: Auto Manual/3(Auto_Gear), ShiftLogic/2(GearNr_[-])  "GearNr_[-]"
  Transmission/2(TransmissionTorque_[Nm]) -> Chassis/1(TransmissionTorque_[Nm])  "TransmissionTorque_[Nm]"
  Transmission/1(ImpellerTorque_[Nm]) -> Engine/1(ImpellerTorque_[Nm])  "ImpellerTorque_[Nm]"
  Gain/1 -> Bus Creator/1  "Vx_[kmh-1]"
  [RPM] -> Bus Creator/2  "NEngine_[rpm]"
  [gear] -> Bus Creator/3  "Gear_[-]"
  [ay] -> Bus Creator/5  "Ay_[ms-2]"
  [auto_manual] -> Bus Creator/6  "Auto_Manual_[-]"
  [throttle] -> Bus Creator/7  "Throttle_[perc]"
  [brake] -> Bus Creator/8  "Brake_[bar]"
  Engine/2(PEngine_[kW]) -> [PE]
  Bus Creator/1 -> Perf_Params/1
  [PE] -> Bus Creator/9  "PEngine_[kW]"
  Radians to Degrees/1 -> Bus Creator/11  "Roll_[deg]"
  Radians to Degrees1/1 -> Bus Creator/12  "Pitch_[deg]"
  [PD] -> Bus Creator/10  "PDrive_[kW]"
  Selector/1 -> Radians to Degrees/1
  Selector1/1 -> Radians to Degrees1/1
  [vx] -> Gain/1
  [ax] -> Bus Creator/4  "Ax_[ms-2]"
  Chassis/8(Out1) -> Out1/1

== system Experiment_134_cs/Ford_Fiesta_Hatchback_1/SELF_Demux ==
  SELF : Inport  OutDataTypeStr=Bus: PRESCAN_SELFSENSORDATA
  Bus Selector : BusSelector  OutputSignals=PositionX,PositionY,PositionZ,OrientationRoll,OrientationPitch,OrientationYaw,Velocity,Yaw_rate,Lat,Long,Alt
  Demux2 : Demux  Outputs=3
  Gain : Gain  Gain=180/pi
  Gain1 : Gain  Gain=180/pi
  Vector Concatenate1 : Concatenate  NumInputs=3
  compas converter : Subsystem
  x [m] : Outport
  y [m] : Outport  Port=2
  z [m] : Outport  Port=3
  rotx [deg] : Outport  Port=4
  roty [deg] : Outport  Port=5
  rotz [deg] : Outport  Port=6
  GPS lat [deg] : Outport  Port=7
  GPS long [deg] : Outport  Port=8
  GPS alt [m] : Outport  Port=9
  velocity [m/s] : Outport  Port=10
  heading [deg] : Outport  Port=11
  yaw rate [deg/s] : Outport  Port=12
  wires:
  Bus Selector/11 -> GPS alt [m]/1  "<Alt>"
  Bus Selector/10 -> GPS long [deg]/1  "<Long>"
  Bus Selector/9 -> GPS lat [deg]/1  "<Lat>"
  Bus Selector/8 -> Gain1/1  "<Yaw_rate>"
  Bus Selector/7 -> velocity [m/s]/1  "<Velocity>"
  Bus Selector/6 -> compas converter/1(rotz [rad]), Vector Concatenate1/3  "<OrientationYaw>"
  Bus Selector/5 -> Vector Concatenate1/2  "<OrientationPitch>"
  Bus Selector/4 -> Vector Concatenate1/1  "<OrientationRoll>"
  Vector Concatenate1/1 -> Gain/1
  Bus Selector/3 -> z [m]/1  "<PositionZ>"
  Bus Selector/2 -> y [m]/1  "<PositionY>"
  Bus Selector/1 -> x [m]/1  "<PositionX>"
  SELF/1 -> Bus Selector/1
  Gain/1 -> Demux2/1
  Demux2/1 -> rotx [deg]/1
  Demux2/2 -> roty [deg]/1
  Demux2/3 -> rotz [deg]/1
  compas converter/1(heading [deg]) -> heading [deg]/1
  Gain1/1 -> yaw rate [deg/s]/1
